simulink library "dcc"  (Simulink 8.1)
settings: Solver=ode1  StartTime=0.0  StopTime=Inf  FixedStep=0.001  RelTol=1e-3
PostLoadFcn:
  | , if any(exist('dsrtsu_mdlpostloadfcn', 'file') == [2, 3, 6]), try dsrtsu_mdlpostloadfcn('Execute', bdroot); catch fprintf('Error in PostLoadFcn (dsrtsu_mdlpostloadfcn) for model "%s":\n %s\n', bdroot, lasterr); end, end,
undefined symbols (not defined in the file or in its folder): FALSE, TRUE
settings Model: DSRTSU_INTERNAL_RTI_VER=450  DSRTSU_INTERNAL_RTI_TYPE=rti1401  RTICANMMDATA=struct('GeneralSetupData',struct('modelroot','D:\ELN150201_TAIWAN\trunk\AdasDragon\software\sw_development\arch\app\acc','generalsettings',struct('filesettings',struct('destfolder',struct('Name','RTICANMM_FILES','Check',1),'buildfolder',struct('Name','.','Check',1),'AbsDestfolder',struct('Name','D:\ELN150201_TAIWAN\trunk\AdasDragon\software\sw_development\arch\app\acc\RTICANMM_FILES'),'AbsBuildfolder',struct('Name','D:\ELN150201_TAIWAN\trunk\AdasDragon\software\sw_development\arch\app\acc'))),'options',struct('addpaths',1,'rmpaths',1,'addtrcexclusion',logical(1),'cannavigator',struct('checkmonitoring',0),'show_usrtrc',0,'use_usrtrc',0),'advanced',struct('options',[1 1 1 1 1 1 1 1 1 1 1 1 1 1 1 1 1 1 1 1 1 1 1 1 1 1 1 1 1 1 1 1 1 1 1 1 1 1 1 1 1 1 1 1 1 1 1 1 1 1 1 1 1 1 1 1 1 1 1 1 1 1 1 1 1 1 1 1 1 1 1 1 1 1 1 1 1 1 1 1 1 1 1 1 1 1 1 1 1 1 1 1 1 1 1 1 1 1 1 1]),'MPSetup',{{}},'modelname','dcc','block','dcc'))  DSRTSU_INTERNAL_RTIFPGA=40  Creator=AT015555  LastModifiedBy=AT015555

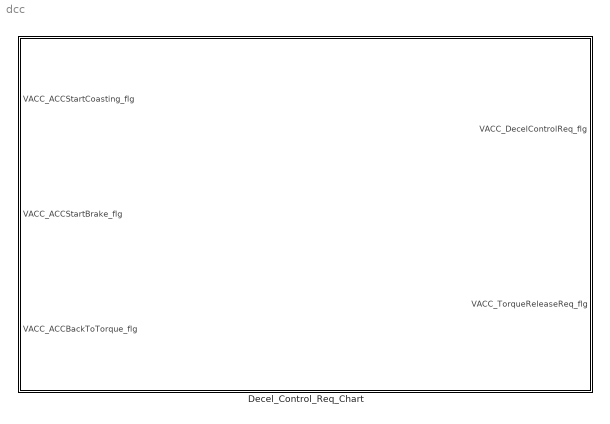
== system dcc ==
  Decel_Control_Req_Chart : Stateflow chart  TreatAsAtomicUnit=on

== stateflow chart Decel_Control_Req_Chart ==
  state NO_BRAKE
    en:
    VACC_DecelControlReq_flg = FALSE;
    VACC_TorqueReleaseReq_flg = FALSE;
  state BRAKE
    en:
    VACC_DecelControlReq_flg = TRUE;
    VACC_TorqueReleaseReq_flg = TRUE;
  state RELEASE
    en:
    VACC_DecelControlReq_flg = FALSE;
    VACC_TorqueReleaseReq_flg = TRUE;
  (default) -> NO_BRAKE
  NO_BRAKE -> RELEASE : [VACC_ACCStartCoasting_flg==TRUE...
      | || VACC_ACCStartBrake_flg ==TRUE]
  RELEASE -> BRAKE [order 2] : [VACC_ACCStartBrake_flg==TRUE]
  RELEASE -> NO_BRAKE [order 1] : [VACC_ACCBackToTorque_flg==TRUE]
  (junction 13) -> NO_BRAKE
  BRAKE -> (junction 14)
  (junction 14) -> (junction 13) : [VACC_ACCBackToTorque_flg==TRUE]
  data: VACC_ACCStartCoasting_flg input double; VACC_DecelControlReq_flg output boolean; VACC_ACCStartBrake_flg input double; VACC_ACCBackToTorque_flg input double; TRUE parameter boolean; FALSE parameter boolean; VACC_TorqueReleaseReq_flg output boolean
